simulink model "reg_observer"  (R2014b)
settings: Solver=ode45  StartTime=0.0  StopTime=10.0  RelTol=1e-3
undefined symbols (not defined in the file): A11, A12, A21, A22, B_1, B_2, L, Tp, x0_observer
settings Model: Creator=Konrad  LastModifiedBy=Konrad

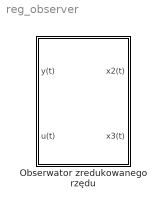
== system reg_observer ==
  Obserwator zredukowanego rzędu : Subsystem

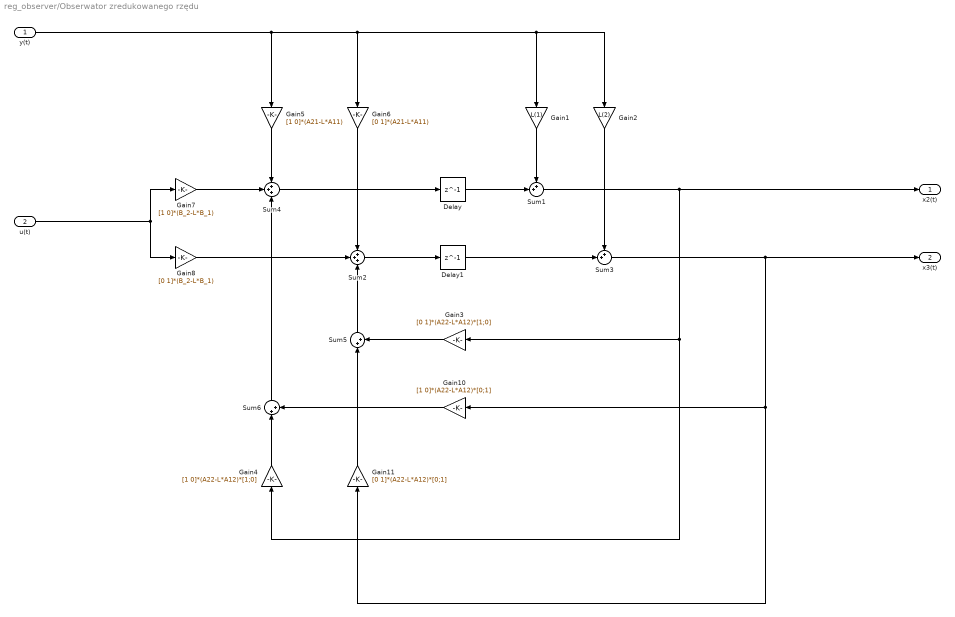
== system reg_observer/Obserwator zredukowanego rzędu ==
  y(t) : Inport
  u(t) : Inport  Port=2
  Delay : Delay  DelayLength=1  InitialCondition=x0_observer(1)  SampleTime=Tp
  Delay1 : Delay  DelayLength=1  InitialCondition=x0_observer(2)  SampleTime=Tp
  Gain1 : Gain  Gain=L(1)
  Gain10 : Gain  Gain=[1 0]*(A22-L*A12)*[0;1]
  Gain11 : Gain  Gain=[0 1]*(A22-L*A12)*[0;1]
  Gain2 : Gain  Gain=L(2)
  Gain3 : Gain  Gain=[0 1]*(A22-L*A12)*[1;0]
  Gain4 : Gain  Gain=[1 0]*(A22-L*A12)*[1;0]
  Gain5 : Gain  Gain=[1 0]*(A21-L*A11)
  Gain6 : Gain  Gain=[0 1]*(A21-L*A11)
  Gain7 : Gain  Gain=[1 0]*(B_2-L*B_1)
  Gain8 : Gain  Gain=[0 1]*(B_2-L*B_1)
  Sum1 : Sum  Inputs=++|
  Sum2 : Sum  Inputs=+++
  Sum3 : Sum  Inputs=++|
  Sum4 : Sum  Inputs=+++
  Sum5 : Sum  Inputs=|++
  Sum6 : Sum  Inputs=|++
  x2(t) : Outport
  x3(t) : Outport  Port=2
  wires:
  Sum6/1 -> Sum4/3
  Sum2/1 -> Delay1/1
  y(t)/1 -> Gain5/1, Gain6/1, Gain2/1, Gain1/1
  Delay/1 -> Sum1/2
  Gain7/1 -> Sum4/2
  Gain2/1 -> Sum3/1
  Sum4/1 -> Delay/1
  Gain6/1 -> Sum2/1
  u(t)/1 -> Gain8/1, Gain7/1
  Sum1/1 -> x2(t)/1, Gain4/1, Gain3/1
  Sum5/1 -> Sum2/3
  Gain1/1 -> Sum1/1
  Gain10/1 -> Sum6/2
  Gain5/1 -> Sum4/1
  Sum3/1 -> x3(t)/1, Gain11/1, Gain10/1
  Gain11/1 -> Sum5/1
  Delay1/1 -> Sum3/2
  Gain3/1 -> Sum5/2
  Gain4/1 -> Sum6/1
  Gain8/1 -> Sum2/2
